simulink library "SimuCopterToolbox"  (R2014a)
settings: Solver=ode45  StartTime=0.0  StopTime=10.0  RelTol=1e-3
libraries: simulink x1
settings Model: Creator=admin  LastModifiedBy=admin

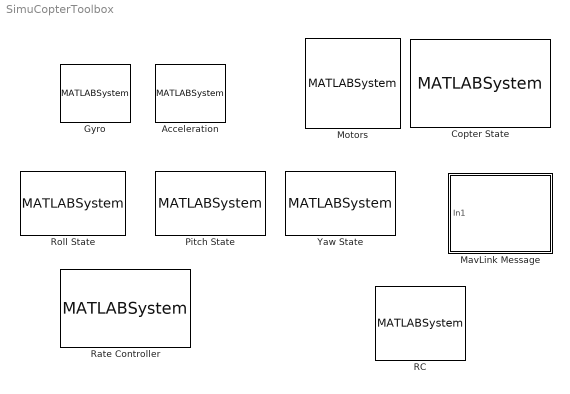
== system SimuCopterToolbox ==
  Acceleration : MATLABSystem  System=Accel
      mask Type: Accel
      mask Display:
      | disp('Accel');
      | port_label('output',1,'x');
      | port_label('output',2,'y');
      | port_label('output',3,'z');
  Copter State : MATLABSystem  System=Copter_Self_State
      mask Type: Copter_Self_State
      mask Display:
      | disp('Copter_Self_State');
      | port_label('output',1,'yaw');
      | port_label('output',2,'roll');
      | port_label('output',3,'pitch');
  Gyro : MATLABSystem  System=Gyro
      mask Type: Gyro
      mask Display:
      | disp('Gyro');
      | port_label('output',1,'x');
      | port_label('output',2,'y');
      | port_label('output',3,'z');
  MavLink Message : Subsystem
  Motors : MATLABSystem  System=Motors
      mask Type: Motors
      mask Display:
      | disp('Motors');
      | port_label('input',1,'roll');
      | port_label('input',2,'pitch');
      | port_label('input',3,'yaw');
      | port_label('input',4,'throttle');
  Pitch State : MATLABSystem  System=Yaw_state
      mask Type: Yaw_state
      mask Display:
      | disp('Yaw_state');
      | port_label('output',1,'yaw');
  RC : MATLABSystem  System=RC
      mask Type: RC
      mask Display:
      | disp('RC');
      | port_label('output',1,'thort');
      | port_label('output',2,'yawR');
      | port_label('output',3,'pitch');
      | port_label('output',4,'roll');
  Rate Controller : MATLABSystem  System=RateController
      mask Type: RateController
      mask Display:
      | disp('RateController');
      | port_label('input',1,'yaw');
      | port_label('input',2,'pitch');
      | port_label('input',3,'roll');
  Roll State : MATLABSystem  System=Roll_state
      mask Type: Roll_state
      mask Display:
      | disp('Roll_state');
      | port_label('output',1,'roll');
  Yaw State : MATLABSystem  System=Pitch_state
      mask Type: Pitch_state
      mask Display:
      | disp('Pitch_state');
      | port_label('output',1,'pitch');

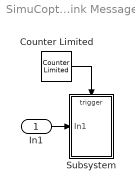
== system SimuCopterToolbox/MavLink Message ==
  In1 : Inport
  Counter Limited : simulink/Sources/Counter Limited  uplimit=100  tsamp=-1
  Subsystem : Subsystem
  wires:
  In1/1 -> Subsystem/1(In1)
  Counter Limited/1 -> Subsystem/Trigger

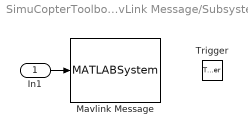
== system SimuCopterToolbox/MavLink Message/Subsystem ==
  In1 : Inport
  Trigger : TriggerPort  PortDimensions=1
  Mavlink Message : MATLABSystem  System=MavlinkMsg  Message=Type a message to send
      mask Type: MavlinkMsg
      mask Display:
      | disp('MavlinkMsg');
      | port_label('input',1,'u');
  wires:
  In1/1 -> Mavlink Message/1
